simulink model "anatoDig"  (R2022b)
settings: Solver=VariableStepAuto  StartTime=0.0  StopTime=10.0  RelTol=1e-3
values from neighbouring files (symbols this model uses):
  h = (2.59/10)    (= 0.259)    [continuoAdiscreto.m]
libraries: cstblocks x4, simulink x2
settings Model: Creator=Lambdax  LastModifiedBy=Lambdax

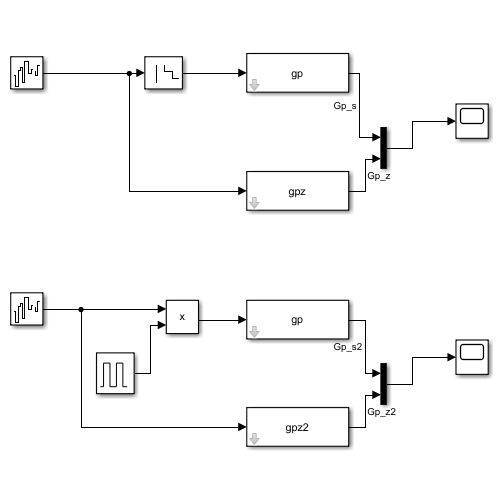
[thumbnail: Simulink's stored preview of the top-level diagram]
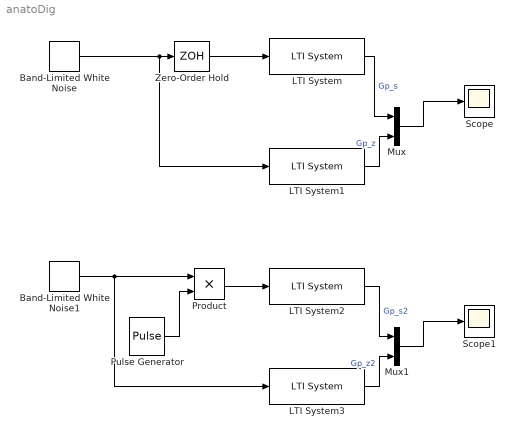
== system anatoDig ==
  Band-Limited White Noise : simulink/Sources/Band-Limited White Noise  Cov=[0.1]  Ts=0.1  seed=[23341]
  Band-Limited White Noise1 : simulink/Sources/Band-Limited White Noise  Cov=[0.1]  Ts=0.1  seed=[23341]
  LTI System : cstblocks/LTI System  sys=gp  IC=[]
  LTI System1 : cstblocks/LTI System  sys=gpz  IC=[]
  LTI System2 : cstblocks/LTI System  sys=gp  IC=[]
  LTI System3 : cstblocks/LTI System  sys=gpz2  IC=[]
  Mux : Mux  Inputs=2
  Mux1 : Mux  Inputs=2
  Product : Product
  Pulse Generator : DiscretePulseGenerator  PulseType=Time based  Amplitude=100/h  Period=h
  Scope : Scope
  Scope1 : Scope
  Zero-Order Hold : ZeroOrderHold  SampleTime=h
  wires:
  Zero-Order Hold/1 -> LTI System/1
  Band-Limited White Noise/1 -> LTI System1/1, Zero-Order Hold/1
  Mux/1 -> Scope/1
  LTI System/1 -> Mux/1  "Gp_s"
  LTI System1/1 -> Mux/2  "Gp_z"
  Mux1/1 -> Scope1/1
  Band-Limited White Noise1/1 -> Product/1, LTI System3/1
  LTI System3/1 -> Mux1/2  "Gp_z2"
  LTI System2/1 -> Mux1/1  "Gp_s2"
  Pulse Generator/1 -> Product/2
  Product/1 -> LTI System2/1
